simulink model "quadrotor_pid_final"  (R2024b)
settings: Solver=ode4  StartTime=0.0  StopTime=100  FixedStep=0.01  RelTol=1e-3
InitFcn:
  | addpath("C:\Users\Administrator\Desktop\stuff\quad")
  | quadrotor_para
values from neighbouring files (symbols this model uses):
  g = 9.81    [quadrotor_para.m]
  Ixx = 1.25    [quadrotor_para.m]
  Iyy = 1.25    [quadrotor_para.m]
  Izz = 1.25    [quadrotor_para.m]
  k1 = 0.01    [quadrotor_para.m]
  k2 = 0.01    [quadrotor_para.m]
  k3 = 0.01    [quadrotor_para.m]
  k4 = 0.012    [quadrotor_para.m]
  k5 = 0.012    [quadrotor_para.m]
  k6 = 0.012    [quadrotor_para.m]
  kd1 = 5    [quadrotor_para.m]
  kd2 = 4    [quadrotor_para.m]
  kd3 = 4    [quadrotor_para.m]
  kd4 = 40    [quadrotor_para.m]
  kd5 = 40    [quadrotor_para.m]
  kd6 = 40    [quadrotor_para.m]
  kp1 = 6    [quadrotor_para.m]
  kp2 = 8    [quadrotor_para.m]
  kp3 = 8    [quadrotor_para.m]
  kp4 = 200    [quadrotor_para.m]
  kp5 = 200    [quadrotor_para.m]
  kp6 = 200    [quadrotor_para.m]
  l = 0.2    [quadrotor_para.m]
  m = 2    [quadrotor_para.m]
libraries: simulink x4, shared6dof x1
settings Model: Creator=zzy  LastModifiedBy=Administrator
settings RTWCC: GPUComputeCapability=3.5

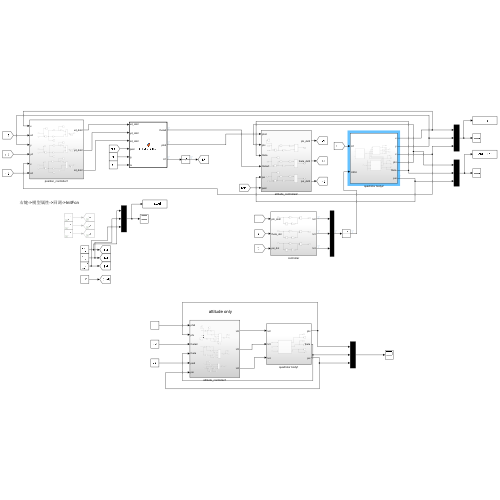
[thumbnail: Simulink's stored preview of the top-level diagram]
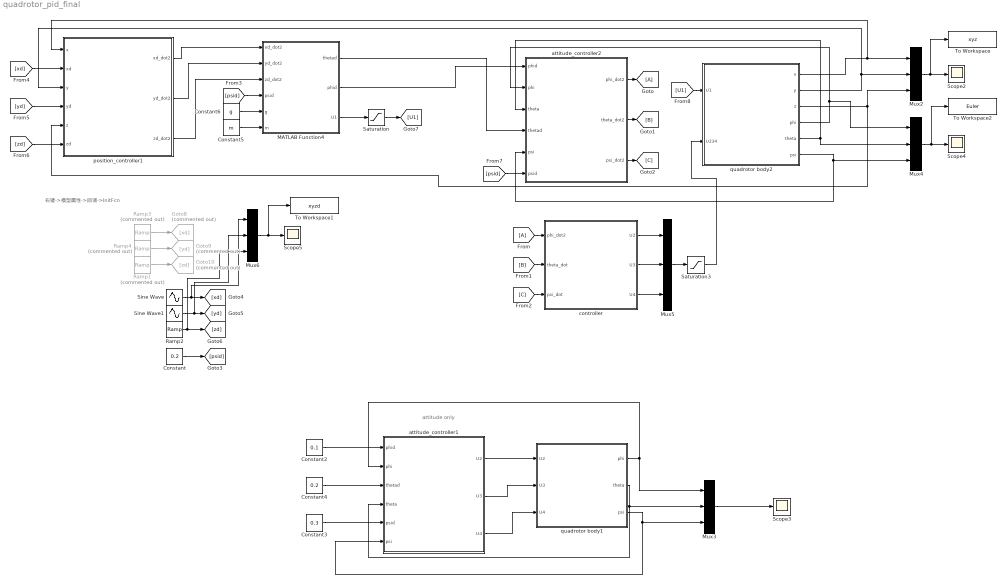
== system quadrotor_pid_final ==
  note: 右键->模型属性->回调->InitFcn
  note: attitude only
  Constant : Constant  Value=0.2
  Constant2 : Constant  Value=0.1
  Constant3 : Constant  Value=0.3
  Constant4 : Constant  Value=0.2
  Constant5 : Constant  Value=m
  Constant6 : Constant  Value=g
  From : From
  Goto : Goto
  Goto10 : Goto  Commented=on  GotoTag=zd
  Goto8 : Goto  Commented=on  GotoTag=xd
  Goto9 : Goto  Commented=on  GotoTag=yd
  MATLAB Function4 : MATLAB Function  TreatAsAtomicUnit=on
  Mux{2..6} (5 alike) : Mux  Inputs=3
  Ramp1 : simulink/Sources/Ramp  Commented=on  slope=0.5  start=0  InitialOutput=0
  Ramp2 : simulink/Sources/Ramp  slope=0.2  start=0  InitialOutput=0
  Ramp3 : simulink/Sources/Ramp  Commented=on  slope=0.1  start=0  InitialOutput=0
  Ramp4 : simulink/Sources/Ramp  Commented=on  slope=0.1  start=0  InitialOutput=0
  Saturation : Saturate  UpperLimit=2.5*m*g  LowerLimit=0
  Saturation3 : Saturate  UpperLimit=10  LowerLimit=-10
  Scope{2..5} (4 alike) : Scope
  Sine Wave : Sin  Amplitude=8  Frequency=0.1  SampleTime=0
  Sine Wave1 : Sin  Amplitude=8  Frequency=0.1  Phase=pi/2  SampleTime=0
  To Workspace : ToWorkspace  VariableName=xyz  SampleTime=-1
  To Workspace1 : ToWorkspace  VariableName=xyzd  SampleTime=-1
  To Workspace2 : ToWorkspace  VariableName=Euler  SampleTime=-1
  attitude_controller1 : Subsystem
  attitude_controller2 : Subsystem
  controller : Subsystem
  position_controller1 : Subsystem
  quadrotor body1 : Subsystem
  quadrotor body2 : Subsystem
  wires:
  attitude_controller1/1(U2) -> quadrotor body1/1(U2)
  quadrotor body1/2(theta) -> attitude_controller1/4(theta), Mux3/2
  quadrotor body1/3(psi) -> attitude_controller1/6(psi), Mux3/3
  Mux3/1 -> Scope3/1
  attitude_controller1/3(U4) -> quadrotor body1/3(U4)
  attitude_controller1/2(U3) -> quadrotor body1/2(U3)
  quadrotor body1/1(phi) -> Mux3/1, attitude_controller1/2(phi)
  Constant2/1 -> attitude_controller1/1(phid)
  Constant3/1 -> attitude_controller1/5(psid)
  Constant4/1 -> attitude_controller1/3(thetad)
  position_controller1/1(xd_dot2) -> MATLAB Function4/1(xd_dot2)
  quadrotor body2/2(y) -> position_controller1/3(y), Mux2/2
  quadrotor body2/6(psi) -> attitude_controller2/5(psi), Mux4/3
  position_controller1/2(yd_dot2) -> MATLAB Function4/2(yd_dot2)
  quadrotor body2/3(z) -> Mux2/3, position_controller1/5(z)
  quadrotor body2/5(theta) -> attitude_controller2/3(theta), Mux4/2
  quadrotor body2/4(phi) -> Mux4/1, attitude_controller2/2(phi)
  quadrotor body2/1(x) -> Mux2/1, position_controller1/1(x)
  Constant5/1 -> MATLAB Function4/6(m)
  Constant6/1 -> MATLAB Function4/5(g)
  Mux2/1 -> To Workspace/1, Scope2/1
  position_controller1/3(zd_dot2) -> MATLAB Function4/3(zd_dot2)
  attitude_controller2/1(phi_dot2) -> Goto/1
  From/1 -> controller/1(phi_dot2)
  attitude_controller2/2(theta_dot2) -> [B]
  attitude_controller2/3(psi_dot2) -> [C]
  [C] -> controller/3(psi_dot)
  [B] -> controller/2(theta_dot)
  controller/1(U2) -> Mux5/1
  controller/2(U3) -> Mux5/2
  [xd] -> position_controller1/2(xd)
  [yd] -> position_controller1/4(yd)
  [zd] -> position_controller1/6(zd)
  [psid] -> MATLAB Function4/4(psid)
  [psid] -> attitude_controller2/6(psid)
  Constant/1 -> [psid]
  [U1] -> quadrotor body2/1(U1)
  MATLAB Function4/1(thetad) -> attitude_controller2/4(thetad)
  MATLAB Function4/2(phid) -> attitude_controller2/1(phid)
  MATLAB Function4/3(U1) -> Saturation/1
  Saturation/1 -> [U1]
  controller/3(U4) -> Mux5/3
  Mux5/1 -> Saturation3/1
  Saturation3/1 -> quadrotor body2/2(U234)
  Sine Wave/1 -> Mux6/1, [xd]
  Sine Wave1/1 -> Mux6/2, [yd]
  Ramp2/1 -> Mux6/3, [zd]
  Ramp3/1 -> Goto8/1
  Ramp4/1 -> Goto9/1
  Ramp1/1 -> Goto10/1
  Mux6/1 -> To Workspace1/1, Scope5/1
  Mux4/1 -> To Workspace2/1, Scope4/1

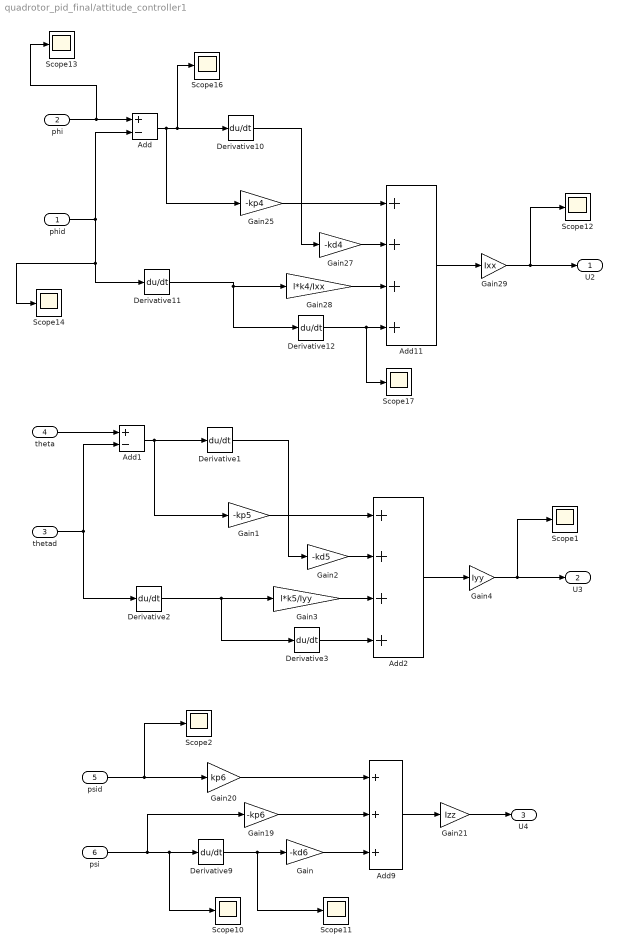
== system quadrotor_pid_final/attitude_controller1 ==
  phid : Inport
  phi : Inport  Port=2
  thetad : Inport  Port=3
  theta : Inport  Port=4
  psid : Inport  Port=5
  psi : Inport  Port=6
  Add : Sum  Inputs=+-
  Add1 : Sum  Inputs=+-
  Add11 : Sum  Inputs=++++
  Add2 : Sum  Inputs=++++
  Add9 : Sum  Inputs=+++
  Derivative{1..3,9..12} (7 alike) : Derivative
  Gain : Gain  Gain=-kd6
  Gain1 : Gain  Gain=-kp5
  Gain19 : Gain  Gain=-kp6
  Gain2 : Gain  Gain=-kd5
  Gain20 : Gain  Gain=kp6
  Gain21 : Gain  Gain=Izz
  Gain25 : Gain  Gain=-kp4
  Gain27 : Gain  Gain=-kd4
  Gain28 : Gain  Gain=l*k4/Ixx
  Gain29 : Gain  Gain=Ixx
  Gain3 : Gain  Gain=l*k5/Iyy
  Gain4 : Gain  Gain=Iyy
  Scope{1..2,10..14,16..17} (9 alike) : Scope
  U2 : Outport
  U3 : Outport  Port=2
  U4 : Outport  Port=3
  wires:
  psi/1 -> Gain19/1, Scope10/1, Derivative9/1
  Derivative9/1 -> Scope11/1, Gain/1
  Gain/1 -> Add9/3
  Gain19/1 -> Add9/2
  Gain20/1 -> Add9/1
  psid/1 -> Scope2/1, Gain20/1
  Add9/1 -> Gain21/1
  Gain21/1 -> U4/1
  Add/1 -> Gain25/1, Derivative10/1, Scope16/1
  Add11/1 -> Gain29/1
  Gain29/1 -> Scope12/1, U2/1
  phi/1 -> Scope13/1, Add/1
  Gain25/1 -> Add11/1
  Gain27/1 -> Add11/2
  Derivative10/1 -> Gain27/1
  phid/1 -> Derivative11/1, Scope14/1, Add/2
  Gain28/1 -> Add11/3
  Derivative11/1 -> Derivative12/1, Gain28/1
  Derivative12/1 -> Scope17/1, Add11/4
  Derivative3/1 -> Add2/4
  Gain3/1 -> Add2/3
  Derivative2/1 -> Derivative3/1, Gain3/1
  Gain2/1 -> Add2/2
  thetad/1 -> Derivative2/1, Add1/2
  theta/1 -> Add1/1
  Gain4/1 -> Scope1/1, U3/1
  Derivative1/1 -> Gain2/1
  Add1/1 -> Derivative1/1, Gain1/1
  Gain1/1 -> Add2/1
  Add2/1 -> Gain4/1

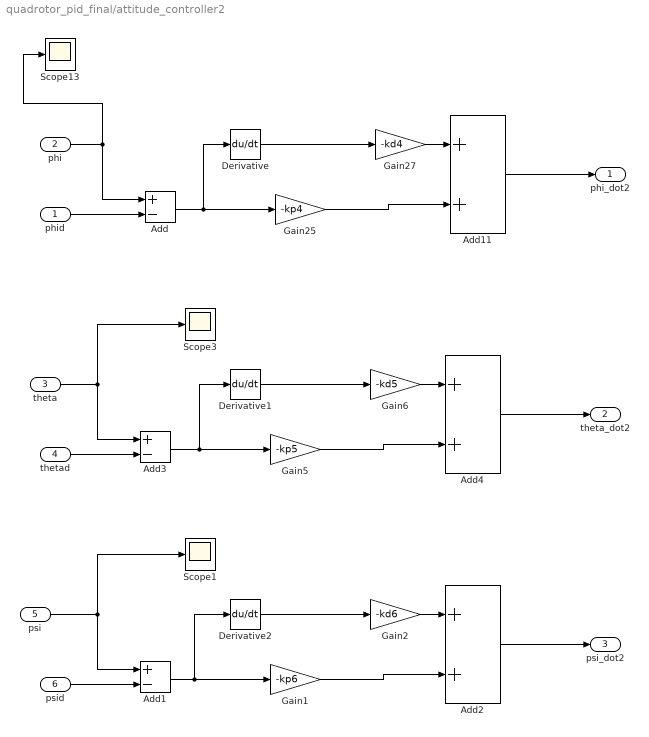
== system quadrotor_pid_final/attitude_controller2 ==
  phid : Inport
  phi : Inport  Port=2
  theta : Inport  Port=3
  thetad : Inport  Port=4
  psi : Inport  Port=5
  psid : Inport  Port=6
  Add : Sum  Inputs=+-
  Add1 : Sum  Inputs=+-
  Add11 : Sum
  Add2 : Sum
  Add3 : Sum  Inputs=+-
  Add4 : Sum
  Derivative : Derivative
  Derivative1 : Derivative
  Derivative2 : Derivative
  Gain1 : Gain  Gain=-kp6
  Gain2 : Gain  Gain=-kd6
  Gain25 : Gain  Gain=-kp4
  Gain27 : Gain  Gain=-kd4
  Gain5 : Gain  Gain=-kp5
  Gain6 : Gain  Gain=-kd5
  Scope1 : Scope
  Scope13 : Scope
  Scope3 : Scope
  phi_dot2 : Outport
  theta_dot2 : Outport  Port=2
  psi_dot2 : Outport  Port=3
  wires:
  Add/1 -> Derivative/1, Gain25/1
  Add11/1 -> phi_dot2/1
  phi/1 -> Add/1, Scope13/1
  Gain27/1 -> Add11/1
  phid/1 -> Add/2
  Gain25/1 -> Add11/2
  Gain5/1 -> Add4/2
  thetad/1 -> Add3/2
  Add3/1 -> Derivative1/1, Gain5/1
  Add4/1 -> theta_dot2/1
  Gain6/1 -> Add4/1
  Add2/1 -> psi_dot2/1
  Add1/1 -> Derivative2/1, Gain1/1
  Derivative2/1 -> Gain2/1
  psi/1 -> Add1/1, Scope1/1
  psid/1 -> Add1/2
  Gain1/1 -> Add2/2
  Gain2/1 -> Add2/1
  Derivative/1 -> Gain27/1
  theta/1 -> Add3/1, Scope3/1
  Derivative1/1 -> Gain6/1

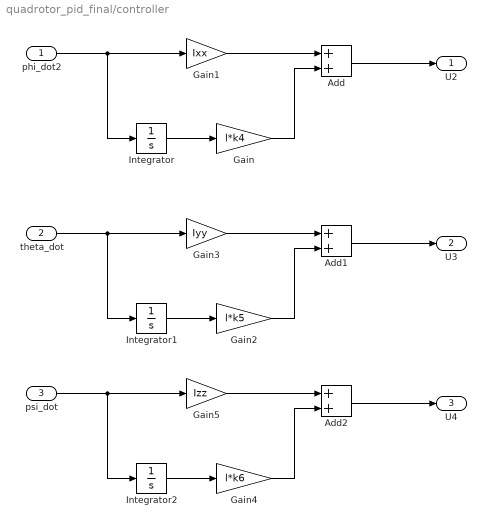
== system quadrotor_pid_final/controller ==
  phi_dot2 : Inport
  theta_dot : Inport  Port=2
  psi_dot : Inport  Port=3
  Add : Sum
  Add1 : Sum
  Add2 : Sum
  Gain : Gain  Gain=l*k4
  Gain1 : Gain  Gain=Ixx
  Gain2 : Gain  Gain=l*k5
  Gain3 : Gain  Gain=Iyy
  Gain4 : Gain  Gain=l*k6
  Gain5 : Gain  Gain=Izz
  Integrator : Integrator
  Integrator1 : Integrator
  Integrator2 : Integrator
  U2 : Outport
  U3 : Outport  Port=2
  U4 : Outport  Port=3
  wires:
  phi_dot2/1 -> Gain1/1, Integrator/1
  Integrator/1 -> Gain/1
  Gain1/1 -> Add/1
  Gain/1 -> Add/2
  Add/1 -> U2/1
  Add1/1 -> U3/1
  Gain3/1 -> Add1/1
  Gain2/1 -> Add1/2
  theta_dot/1 -> Gain3/1, Integrator1/1
  Integrator1/1 -> Gain2/1
  Add2/1 -> U4/1
  Gain5/1 -> Add2/1
  Gain4/1 -> Add2/2
  psi_dot/1 -> Gain5/1, Integrator2/1
  Integrator2/1 -> Gain4/1

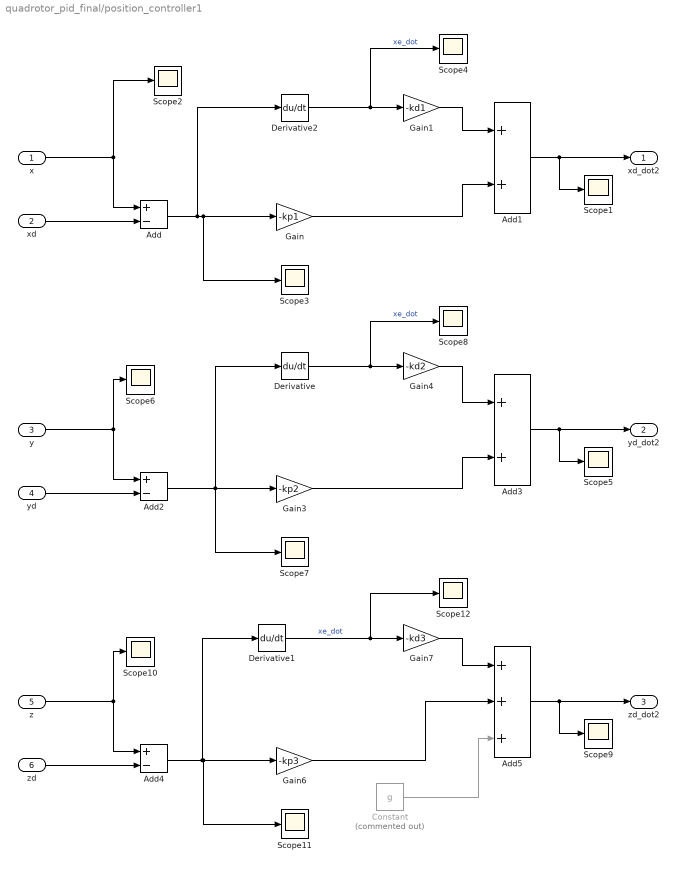
== system quadrotor_pid_final/position_controller1 ==
  x : Inport
  xd : Inport  Port=2
  y : Inport  Port=3
  yd : Inport  Port=4
  z : Inport  Port=5
  zd : Inport  Port=6
  Add : Sum  Inputs=+-
  Add1 : Sum
  Add2 : Sum  Inputs=+-
  Add3 : Sum
  Add4 : Sum  Inputs=+-
  Add5 : Sum  Inputs=+++
  Constant : Constant  Commented=on  Value=g
  Derivative : Derivative
  Derivative1 : Derivative
  Derivative2 : Derivative
  Gain : Gain  Gain=-kp1
  Gain1 : Gain  Gain=-kd1
  Gain3 : Gain  Gain=-kp2
  Gain4 : Gain  Gain=-kd2
  Gain6 : Gain  Gain=-kp3
  Gain7 : Gain  Gain=-kd3
  Scope{1..12} (12 alike) : Scope
  xd_dot2 : Outport
  yd_dot2 : Outport  Port=2
  zd_dot2 : Outport  Port=3
  wires:
  x/1 -> Scope2/1, Add/1
  xd/1 -> Add/2
  Add/1 -> Derivative2/1, Scope3/1, Gain/1
  Derivative2/1 -> Scope4/1, Gain1/1  "xe_dot"
  Add1/1 -> xd_dot2/1, Scope1/1
  Gain1/1 -> Add1/1
  Gain/1 -> Add1/2
  Gain3/1 -> Add3/2
  Gain4/1 -> Add3/1
  yd/1 -> Add2/2
  y/1 -> Add2/1, Scope6/1
  Add3/1 -> yd_dot2/1, Scope5/1
  Add2/1 -> Scope7/1, Gain3/1, Derivative/1
  Derivative/1 -> Gain4/1, Scope8/1  "xe_dot"
  Gain6/1 -> Add5/2
  Gain7/1 -> Add5/1
  zd/1 -> Add4/2
  z/1 -> Scope10/1, Add4/1
  Add5/1 -> zd_dot2/1, Scope9/1
  Add4/1 -> Derivative1/1, Scope11/1, Gain6/1
  Derivative1/1 -> Gain7/1, Scope12/1  "xe_dot"
  Constant/1 -> Add5/3

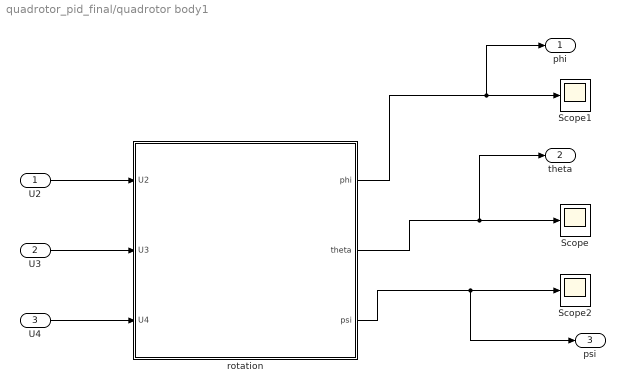
== system quadrotor_pid_final/quadrotor body1 ==
  U2 : Inport
  U3 : Inport  Port=2
  U4 : Inport  Port=3
  Scope : Scope
  Scope1 : Scope
  Scope2 : Scope
  rotation : Subsystem
  phi : Outport
  theta : Outport  Port=2
  psi : Outport  Port=3
  wires:
  rotation/1(phi) -> phi/1, Scope1/1
  rotation/3(psi) -> psi/1, Scope2/1
  U4/1 -> rotation/3(U4)
  rotation/2(theta) -> theta/1, Scope/1
  U2/1 -> rotation/1(U2)
  U3/1 -> rotation/2(U3)

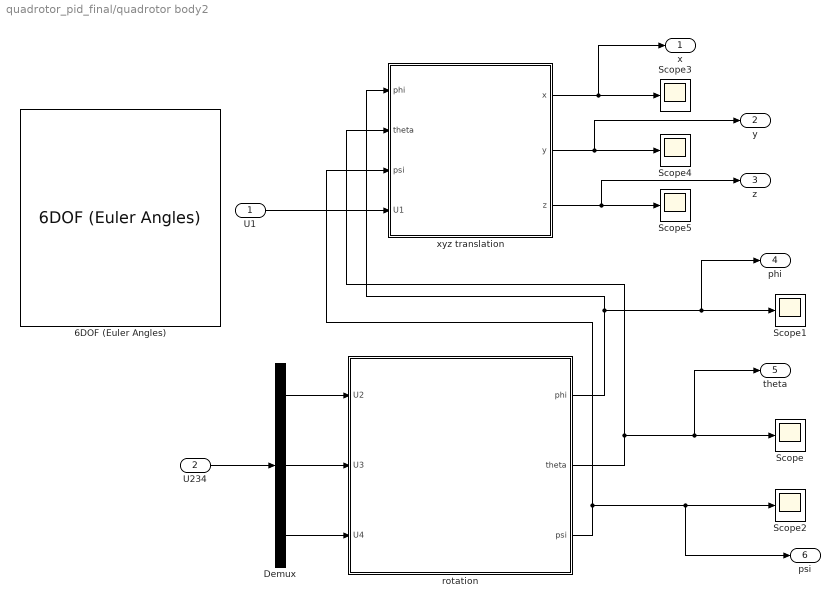
== system quadrotor_pid_final/quadrotor body2 ==
  U1 : Inport
  U234 : Inport  Port=2
  6DOF (Euler Angles) : shared6dof/6DOF (Euler Angles)  units=Metric (MKS)  mtype=Fixed  rep=Euler Angles  xme_0=[0 0 0]  Vm_0=[0 0 0]  eul_0=[0 0 0]  pm_0=[0 0 0]  mass_0=1.0  mass_e=0.5  mass_f=2.0  inertia=eye(3)  inertia_e=eye(3)  inertia_f=2*eye(3)  k_quat=1.0  vre_flag=on  abi_flag=off  aMode=0  xme_statename=''  Vm_statename=''  eul_statename=''  quat_statename=''  pm_statename=''  mass_statename=''
  Demux : Demux  Outputs=3
  Scope{,1..5} (6 alike) : Scope
  rotation : Subsystem
  xyz translation : Subsystem
  x : Outport
  y : Outport  Port=2
  z : Outport  Port=3
  phi : Outport  Port=4
  theta : Outport  Port=5
  psi : Outport  Port=6
  wires:
  rotation/1(phi) -> phi/1, Scope1/1, xyz translation/1(phi)
  xyz translation/1(x) -> x/1, Scope3/1
  rotation/3(psi) -> xyz translation/3(psi), psi/1, Scope2/1
  Demux/3 -> rotation/3(U4)
  rotation/2(theta) -> xyz translation/2(theta), theta/1, Scope/1
  xyz translation/2(y) -> y/1, Scope4/1
  xyz translation/3(z) -> z/1, Scope5/1
  Demux/2 -> rotation/2(U3)
  U1/1 -> xyz translation/4(U1)
  Demux/1 -> rotation/1(U2)
  U234/1 -> Demux/1

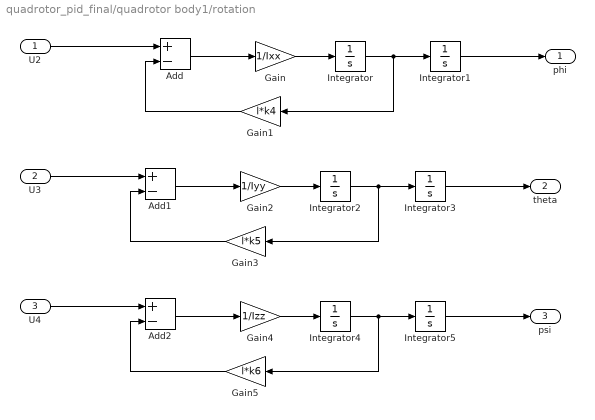
== system quadrotor_pid_final/quadrotor body1/rotation ==
  U2 : Inport
  U3 : Inport  Port=2
  U4 : Inport  Port=3
  Add : Sum  Inputs=+-
  Add1 : Sum  Inputs=+-
  Add2 : Sum  Inputs=+-
  Gain : Gain  Gain=1/Ixx
  Gain1 : Gain  Gain=l*k4
  Gain2 : Gain  Gain=1/Iyy
  Gain3 : Gain  Gain=l*k5
  Gain4 : Gain  Gain=1/Izz
  Gain5 : Gain  Gain=l*k6
  Integrator{,1..5} (6 alike) : Integrator
  phi : Outport
  theta : Outport  Port=2
  psi : Outport  Port=3
  wires:
  Integrator/1 -> Gain1/1, Integrator1/1
  Integrator1/1 -> phi/1
  Add/1 -> Gain/1
  Gain/1 -> Integrator/1
  U2/1 -> Add/1
  Gain1/1 -> Add/2
  Gain2/1 -> Integrator2/1
  Integrator3/1 -> theta/1
  U3/1 -> Add1/1
  Gain3/1 -> Add1/2
  Integrator2/1 -> Gain3/1, Integrator3/1
  Add1/1 -> Gain2/1
  Gain4/1 -> Integrator4/1
  Integrator5/1 -> psi/1
  U4/1 -> Add2/1
  Gain5/1 -> Add2/2
  Integrator4/1 -> Gain5/1, Integrator5/1
  Add2/1 -> Gain4/1

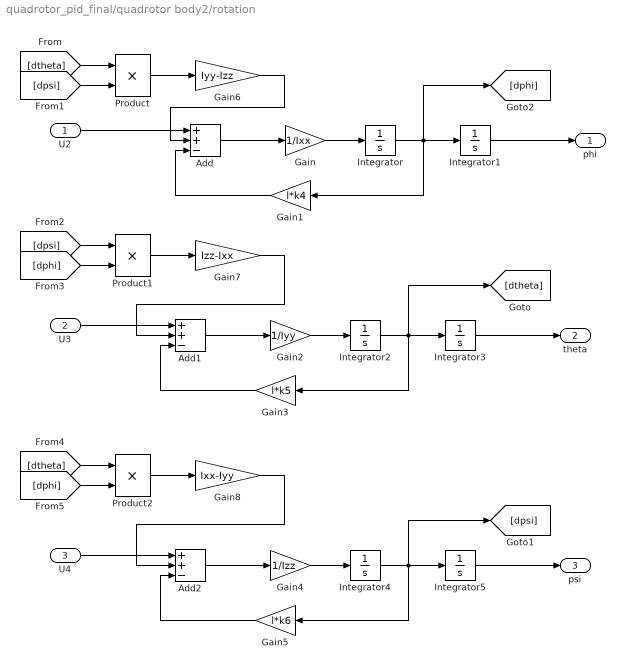
== system quadrotor_pid_final/quadrotor body2/rotation ==
  U2 : Inport
  U3 : Inport  Port=2
  U4 : Inport  Port=3
  Add : Sum  Inputs=++-
  Add1 : Sum  Inputs=++-
  Add2 : Sum  Inputs=++-
  Gain : Gain  Gain=1/Ixx
  Gain1 : Gain  Gain=l*k4
  Gain2 : Gain  Gain=1/Iyy
  Gain3 : Gain  Gain=l*k5
  Gain4 : Gain  Gain=1/Izz
  Gain5 : Gain  Gain=l*k6
  Gain6 : Gain  Gain=Iyy-Izz
  Gain7 : Gain  Gain=Izz-Ixx
  Gain8 : Gain  Gain=Ixx-Iyy
  Integrator{,1..5} (6 alike) : Integrator
  Product : Product
  Product1 : Product
  Product2 : Product
  phi : Outport
  theta : Outport  Port=2
  psi : Outport  Port=3
  wires:
  Integrator1/1 -> phi/1
  Add/1 -> Gain/1
  Gain/1 -> Integrator/1
  U2/1 -> Add/1
  Gain1/1 -> Add/3
  Gain2/1 -> Integrator2/1
  Integrator3/1 -> theta/1
  U3/1 -> Add1/1
  Integrator2/1 -> Integrator3/1, [dtheta], Gain3/1
  Add1/1 -> Gain2/1
  Gain4/1 -> Integrator4/1
  Integrator5/1 -> psi/1
  U4/1 -> Add2/1
  Add2/1 -> Gain4/1
  Product/1 -> Gain6/1
  Integrator4/1 -> [dpsi], Integrator5/1, Gain5/1
  Integrator/1 -> [dphi], Gain1/1, Integrator1/1
  Gain3/1 -> Add1/3
  [dtheta] -> Product/1
  [dpsi] -> Product/2
  Gain6/1 -> Add/2
  Gain7/1 -> Add1/2
  [dpsi] -> Product1/1
  [dphi] -> Product1/2
  Product1/1 -> Gain7/1
  Product2/1 -> Gain8/1
  [dtheta] -> Product2/1
  [dphi] -> Product2/2
  Gain8/1 -> Add2/2
  Gain5/1 -> Add2/3

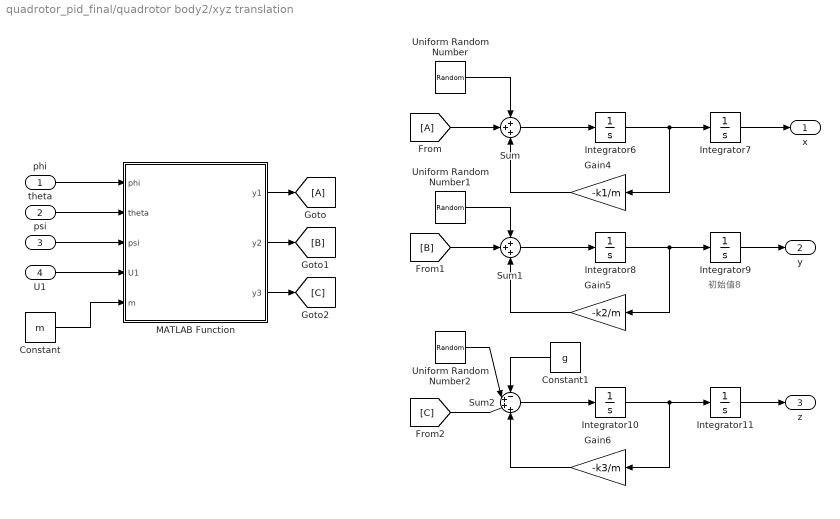
== system quadrotor_pid_final/quadrotor body2/xyz translation ==
  note: 初始值8
  phi : Inport
  theta : Inport  Port=2
  psi : Inport  Port=3
  U1 : Inport  Port=4
  Constant : Constant  Value=m
  Constant1 : Constant  Value=g
  From : From
  Gain4 : Gain  Gain=-k1/m
  Gain5 : Gain  Gain=-k2/m
  Gain6 : Gain  Gain=-k3/m
  Goto : Goto
  Integrator{6..8,10..11} (5 alike) : Integrator
  Integrator9 : Integrator  InitialCondition=8
  MATLAB Function : MATLAB Function  TreatAsAtomicUnit=on
  Sum : Sum  Inputs=+++
  Sum1 : Sum  Inputs=+++
  Sum2 : Sum  Inputs=-+++
  Uniform Random Number : UniformRandomNumber  SampleTime=0.1
  Uniform Random Number1 : UniformRandomNumber  SampleTime=0.1
  Uniform Random Number2 : UniformRandomNumber  SampleTime=0.1
  x : Outport
  y : Outport  Port=2
  z : Outport  Port=3
  wires:
  phi/1 -> MATLAB Function/1(phi)
  theta/1 -> MATLAB Function/2(theta)
  psi/1 -> MATLAB Function/3(psi)
  U1/1 -> MATLAB Function/4(U1)
  MATLAB Function/1(y1) -> Goto/1
  MATLAB Function/2(y2) -> [B]
  MATLAB Function/3(y3) -> [C]
  Integrator6/1 -> Gain4/1, Integrator7/1
  From/1 -> Sum/2
  Sum/1 -> Integrator6/1
  Gain4/1 -> Sum/3
  Integrator7/1 -> x/1
  Integrator9/1 -> y/1
  Gain5/1 -> Sum1/3
  [B] -> Sum1/2
  Sum1/1 -> Integrator8/1
  Integrator8/1 -> Gain5/1, Integrator9/1
  Integrator11/1 -> z/1
  Gain6/1 -> Sum2/4
  Sum2/1 -> Integrator10/1
  Integrator10/1 -> Gain6/1, Integrator11/1
  Constant/1 -> MATLAB Function/5(m)
  Constant1/1 -> Sum2/1
  Uniform Random Number/1 -> Sum/1
  Uniform Random Number1/1 -> Sum1/1
  [C] -> Sum2/3
  Uniform Random Number2/1 -> Sum2/2

== matlab function quadrotor_pid_final/MATLAB Function4 ==
  data: xd_dot2 input; thetad output; phid output; U1 output; yd_dot2 input; zd_dot2 input; psid input; g input; m input
function [thetad, phid, U1]   = attitude_solver(xd_dot2, yd_dot2, zd_dot2, psid, g, m)


if zd_dot2+g > 0
    U1 = sqrt(abs((m*xd_dot2)^2+(m*yd_dot2)^2+(m*zd_dot2+m*g)^2));
else
    U1 = -sqrt(abs((m*xd_dot2)^2+(m*yd_dot2)^2+(m*zd_dot2+m*g)^2));
end


if m*xd_dot2*sin(psid)-m*yd_dot2*cos(psid) > 0
    phid = asin(sqrt((m*xd_dot2*sin(psid)-m*yd_dot2*cos(psid))^2/U1^2));
else
    phid = -asin(sqrt(((m*xd_dot2*sin(psid)-m*yd_dot2*cos(psid))^2)/U1^2));
end

if m*xd_dot2/U1 - sin(phid)*sin(psid) > 0
    thetad = acos(sqrt((m*zd_dot2+m*g)^2/((m*xd_dot2*cos(psid)+m*yd_dot2*sin(psid))^2+(m*zd_dot2+m*g)^2)));
else
    thetad = -acos(sqrt((m*zd_dot2+m*g)^2/((m*xd_dot2*cos(psid)+m*yd_dot2*sin(psid))^2+(m*zd_dot2+m*g)^2)));
end

== matlab function quadrotor_pid_final/quadrotor body2/xyz translation/MATLAB Function ==
  data: phi input; y1 output; theta input; psi input; y2 output; y3 output; U1 input; m input
function [y1, y2, y3] = fcn(phi, theta, psi, U1, m)

y1 = (cos(phi)*sin(theta)*cos(phi) + sin(phi)*sin(psi))*U1/m;

y2 = (cos(phi)*sin(theta)*sin(psi) - sin(phi)*cos(psi))*U1/m;

y3 = (cos(phi)*cos(theta))*U1/m;
